simulink model "First_HIL_Scenario2"  (R2023a)
settings: Solver=ode1  StartTime=0.0  StopTime=inf  FixedStep=0.001  RelTol=1e-3
undefined symbols (not defined in the file or in its folder): ACC_X, ACC_Y, ACC_Z, Altitude, distance, GetTimeDemo, Gyro_X, Gyro_Y, Gyro_Z, Heading, Lane_Car_Distance_Left, Lane_Car_Distance_Right, Lane_Class, Lane_Coefficient_C0, Lane_Coefficient_C1, Lane_Coefficient_C2, Lane_Coefficient_C3, Lane_Curvature, Lane_Distance, Lane_ID, Latitude, Longitude, OBJ_Class, OBJ_Height, OBJ_ID, OBJ_Length, OBJ_RCS, OBJ_S_Azimuth, OBJ_S_Elevation, OBJ_S_Range, OBJ_S_Velocity, OBJ_Velocity, OBJ_Width, OBJ_X, OBJ_Y, OBJ_Z, Pitch, Roll, Subsystem, time, Timestamp, TrafficLight_Direction, TrafficLight_State, TrafficLight_Timer, Velocity, width, x, x1, x2, x3, x4, y, y1, y2, y3, y4, Yaw
(part 3 of 4)

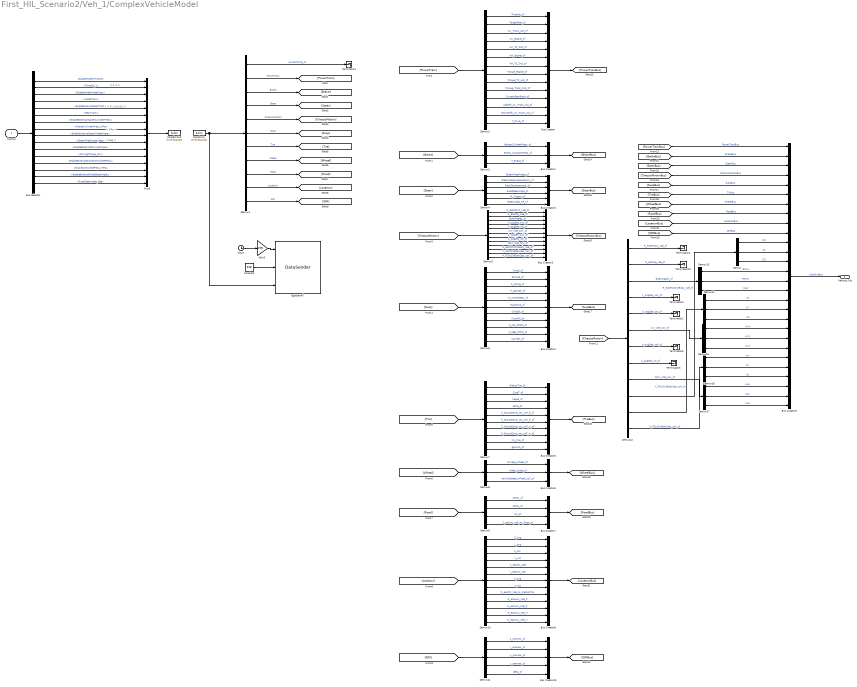
== system First_HIL_Scenario2/Veh_1/ComplexVehicleModel ==
  note: /* MPa */
  note: /* R:-1,N:0,D:1 */
  note: /* 0~1 */
  note: /* Deg */
  Control : Inport
  Bus Creator : BusCreator  Inputs=14
  Bus Creator1 : BusCreator  Inputs=3
  Bus Creator10 : BusCreator  Inputs=5
  Bus Creator2 : BusCreator  Inputs=6
  Bus Creator3 : BusCreator  Inputs=12
  Bus Creator4 : BusCreator  Inputs=11
  Bus Creator5 : BusCreator  Inputs=10
  Bus Creator6 : BusCreator  Inputs=3
  Bus Creator7 : BusCreator  Inputs=4
  Bus Creator8 : BusCreator  Inputs=13
  Bus Creator9 : BusCreator  Inputs=28
  Bus Selector : BusSelector  OutputSignals=EnableModelThrottle,Throttle_1,EnableModelModeTrans,ModeTrans,EnableExternalGearTrans,GearTrans,EnableExternalMasterCylinderPress,MasterCylinderPress_MPa,EnableExternalSteerWheelAngle,SteerWheelAngle_deg,EnableExternalDrivingTorque,DrivingTorque_Nm,EnableExternalBrakeControlledPress,BrakeControlledPress_MPa,EnableExternalRoadSteerAngle,RoadSteerAngle_deg
  Clock : Clock
  Constant : Constant  Value=228  OutDataTypeStr=int32
  Demux{,13..17} (6 alike) : Demux  Outputs=3
  Demux1 : Demux  Outputs=[1 17 9 15 36 42 36 12 16 39 5]
  Demux10 : Demux  Outputs=[1 1 4 4 4 4 1 4 4 3 3 3 3]
  Demux11 : Demux  Outputs=[1 1 1 1 1]
  Demux12 : Demux  Outputs=[3 3 3 3 3 3 3 3 3 3 3 3]
  Demux2 : Demux  Outputs=[1 1 1 1 1 1 1 1 1 1 1 1 1 4]
  Demux3 : Demux  Outputs=[1 4 4]
  Demux4 : Demux  Outputs=[1 1 1 4 4 4]
  Demux5 : Demux  Outputs=[3 3 3 3 3 3 3 3 3 3 3 3]
  Demux6 : Demux  Outputs=[4 4 4 4 2 4 4 4 4 4 4]
  Demux7 : Demux  Outputs=[4 4 4 4 3 3 3 3 4 4]
  Demux8 : Demux  Outputs=[4 4 4]
  Demux9 : Demux  Outputs=[4 4 4 4]
  EgoDataAll : S-Function  FunctionName=DataSender  Parameters='ego_all','time@i,228@[,data@d','0.01','0.0','192.168.2.101','25004'  SFunctionDeploymentMode=off  EnableBusSupport=off
  Gain3 : Gain  Gain=1000  OutDataTypeStr=Inherit: Inherit via back propagation  RndMeth=Nearest
  Mux5 : Mux  Inputs=16
  PanoSimIn : S-Function  Priority=1  FunctionName=NIVeriStandIO  Parameters=width dtype portnum stime stype btype  SFunctionDeploymentMode=off  EnableBusSupport=off  mask(NI VeriStand Inport){portnum=1, width=-1, stime=-1, dtype=auto, stype=auto, btype=1}
      mask prompts: portnum "Port number:"; width "Port dimensions (-1 for dynamically sized):"; stime "Sample time (-1 for inherited):"; dtype "Data type:"; stype "Signal type:"; btype "Block type:"
      mask help: Use this inport on any level of nested subsystems to allow NI VeriStand software to map signals to it.
      mask init:
      | NIVeriStandIO_init;
      settings: CopyFcn=NIVeriStand_MDL_functions('', 'IO_copy');  DeleteFcn=NIVeriStand_MDL_functions('', 'IO_delete');  MoveFcn=set_param(gcb, 'Mask', 'on');
      mask Callback portnum: NIVeriStand_MDL_functions('', 'IO_setportnum');
      mask TypeOptions dtype: auto | double | single | int8 | uint8 | int16 | uint16 | int32 | uint32 | boolean
      mask Callback dtype: NIVeriStand_MDL_functions('', 'IO_booleansignal');
      mask TypeOptions stype: auto | real | complex
      mask Display:
      | patch([-x x], [-y y], [.90980 .81960 .32156]);
      | plot([xrad -x x xrad], [yrad -y y yrad]);
      | fprintf('NI In%d', portnum);
  PanoSimOut : S-Function  Priority=1  FunctionName=NIVeriStandIO  Parameters=width dtype portnum stime stype btype  SFunctionDeploymentMode=off  EnableBusSupport=off  mask(NI VeriStand Outport){portnum=1, width=-1, stime=-1, dtype=auto, stype=auto, btype=0}
      mask prompts: portnum "Port number:"; width "Port dimensions (-1 for dynamically sized):"; stime "Sample time (-1 for inherited):"; dtype "Data type:"; stype "Signal type:"; btype "Block type:"
      mask help: Use this outport on any level of nested subsystems to allow NI VeriStand software to map signals to it.
      mask init:
      | NIVeriStandIO_init;
      settings: CopyFcn=NIVeriStand_MDL_functions('', 'IO_copy');  DeleteFcn=NIVeriStand_MDL_functions('', 'IO_delete');  MoveFcn=set_param(gcb, 'Mask', 'on');
      mask Callback portnum: NIVeriStand_MDL_functions('', 'IO_setportnum');
      mask TypeOptions dtype: auto | double | single | int8 | uint8 | int16 | uint16 | int32 | uint32 | boolean
      mask Callback dtype: NIVeriStand_MDL_functions('', 'IO_booleansignal');
      mask TypeOptions stype: auto | real | complex
      mask Display:
      | patch([-x x], [-y y], [.90980 .81960 .32156]);
      | plot([xrad -x x xrad], [yrad -y y yrad]);
      | fprintf('NI Out%d', portnum);
  Terminator{1..6,20} (7 alike) : Terminator
  Vehicle_Out : Outport
  wires:
  Demux12/4 -> Terminator5/1  "V_scg2eo_coV_sf"
  Demux12/7 -> Terminator6/1  "A_scg2eo_coV_sf"
  Demux12/12 -> Demux16/1  "A_FCtcCinBody2eo_coV_sf"
  Demux12/1 -> Terminator4/1  "R_eo2FCtcC_coE_sf"
  Demux12/11 -> Demux14/1  "V_FCtcCinBody2eo_coV_sf"
  Demux12/10 -> Demux/1  "R_eo2FCtcCinBody_coE_sf"
  Demux12/9 -> Demux17/1  "DAV_V2E_coV_sf"
  Demux12/8 -> Terminator3/1  "A_acg2eo_coI_sf"
  Demux12/3 -> Demux13/1  "EulerAngles_sf"
  Demux12/6 -> Demux15/1  "AV_V2E_coV_sf"
  Demux12/2 -> Terminator20/1  "R_eo2scg_coE_sf"
  Demux12/5 -> Terminator2/1  "V_acg2eo_coI_sf"
  [ChassisMotion] -> Demux12/1
  Demux5/10 -> Bus Creator3/10  "R_eo2FCtcCinBody_coE_sf"
  Demux5/6 -> Bus Creator3/6  "AV_V2E_coV_sf"
  Demux5/3 -> Bus Creator3/3  "EulerAngles_sf"
  Demux5/1 -> Bus Creator3/1  "R_eo2FCtcC_coE_sf"
  Demux5/5 -> Bus Creator3/5  "V_acg2eo_coI_sf"
  Demux5/9 -> Bus Creator3/9  "DAV_V2E_coV_sf"
  Demux5/11 -> Bus Creator3/11  "V_FCtcCinBody2eo_coV_sf"
  Demux5/7 -> Bus Creator3/7  "A_scg2eo_coV_sf"
  Demux5/8 -> Bus Creator3/8  "A_acg2eo_coI_sf"
  Demux5/4 -> Bus Creator3/4  "V_scg2eo_coV_sf"
  Demux5/2 -> Bus Creator3/2  "R_eo2scg_coE_sf"
  Demux5/12 -> Bus Creator3/12  "A_FCtcCinBody2eo_coV_sf"
  Bus Creator3/1 -> [ChassisMotionBus]
  [ChassisMotion] -> Demux5/1
  Demux17/3 -> Bus Creator9/28  "AAz"
  Demux17/2 -> Bus Creator9/27  "AAy"
  Demux17/1 -> Bus Creator9/26  "AAx"
  Demux16/3 -> Bus Creator9/25  "Az"
  Demux16/2 -> Bus Creator9/24  "Ay"
  Demux16/1 -> Bus Creator9/23  "Ax"
  Demux15/3 -> Bus Creator9/22  "AVz"
  Demux15/2 -> Bus Creator9/21  "AVy"
  Demux15/1 -> Bus Creator9/20  "AVx"
  Demux14/3 -> Bus Creator9/19  "VZ"
  Demux14/2 -> Bus Creator9/18  "VY"
  Demux14/1 -> Bus Creator9/17  "VX"
  Demux13/3 -> Bus Creator9/16  "YAW"
  Demux13/2 -> Bus Creator9/15  "PITCH"
  Demux13/1 -> Bus Creator9/14  "ROLL"
  Demux/3 -> Bus Creator9/13  "ZO"
  Demux/2 -> Bus Creator9/12  "YO"
  Demux/1 -> Bus Creator9/11  "XO"
  Demux10/10 -> Bus Creator8/10  "R_eo2uwc_coE_fl"
  Demux6/10 -> Bus Creator4/10  "F_REB_STOP_sf"
  Demux2/9 -> Bus Creator/9  "Torque_TC_out_sf"
  [TireBus] -> Bus Creator9/6  "TirBus"
  Demux4/1 -> Bus Creator2/1  "SteerWheelAngle_sf"
  Demux6/9 -> Bus Creator4/9  "F_JNC_STOP_sf"
  Demux7/6 -> Bus Creator5/6  "F_Ground2tire_ctc_coT_fr_sf"
  Demux2/2 -> Bus Creator/2  "TargetGear_sf"
  Demux9/1 -> Bus Creator7/1  "DZDX_sf"
  [WheelBus] -> Bus Creator9/7  "WheelBus"
  Bus Creator5/1 -> [TireBus]
  Demux7/3 -> Bus Creator5/3  "kappa_sf"
  Demux6/2 -> Bus Creator4/2  "DCmpS_sf"
  Demux7/10 -> Bus Creator5/10  "gamma_sf"
  Bus Creator1/1 -> [BrakeBus]
  Demux4/4 -> Bus Creator2/4  "RoadSteerAngle_sf"
  Demux7/1 -> Bus Creator5/1  "RadiusTire_sf"
  Demux6/11 -> Bus Creator4/11  "Camber_sf"
  Demux4/6 -> Bus Creator2/6  "SteerAngle_KP_sf"
  [Steer] -> Demux4/1
  [BrakeBus] -> Bus Creator9/2  "BrakeBus"
  Demux10/5 -> Bus Creator8/5  "X_eo2ctc_coE"
  Demux6/8 -> Bus Creator4/8  "CmpRSt_sf"
  Demux8/2 -> Bus Creator6/2  "wheel_state_sf"
  Bus Creator7/1 -> [RoadBus]
  Demux2/6 -> Bus Creator/6  "AA_Engine_sf"
  Bus Creator9/1 -> Vehicle_Out/1  "xCarOutBus"
  Demux6/6 -> Bus Creator4/6  "SuspCmp_sf"
  Demux7/7 -> Bus Creator5/7  "F_Ground2tire_ctc_coT_rl_sf"
  Demux2/1 -> Bus Creator/1  "Throttle_sf"
  Demux6/3 -> Bus Creator4/3  "F_spring_sf"
  Demux10/12 -> Bus Creator8/12  "R_eo2uwc_coE_rl"
  Demux4/5 -> Bus Creator2/5  "M_Kingpin_sf"
  Bus Creator10/1 -> [IDMBus]
  Demux2/13 -> Bus Creator/13  "DownShift_AV_Trans_out_sf"
  [Tire] -> Demux7/1
  [PowerTrainBus] -> Bus Creator9/1  "PowerTrainBus"
  Demux3/2 -> Bus Creator1/2  "Brake_ActuatorPress_sf"
  Demux9/2 -> Bus Creator7/2  "DZDY_sf"
  Bus Creator4/1 -> [SuspBus]
  Demux7/9 -> Bus Creator5/9  "My_tire_sf"
  Demux6/5 -> Bus Creator4/5  "M_AntiRollBar_sf"
  Bus Creator/1 -> [PowerTrainBus]
  Demux3/3 -> Bus Creator1/3  "T_Brake_sf"
  Demux2/7 -> Bus Creator/7  "AA_TC_Out_sf"
  Demux2/10 -> Bus Creator/10  "Torque_Trans_Out_sf"
  [PowerTrain] -> Demux2/1
  Demux2/12 -> Bus Creator/12  "UpShift_AV_Trans_out_sf"
  [LocationBus] -> Bus Creator9/9  "LocationBus"
  Demux2/14 -> Bus Creator/14  "T_Drive_sf"
  Demux4/3 -> Bus Creator2/3  "RackDisplacement_sf"
  Demux2/8 -> Bus Creator/8  "Torque_Engine_sf"
  Demux3/1 -> Bus Creator1/1  "MasterCylinderPress_sf"
  [Brake] -> Demux3/1
  Demux10/13 -> Bus Creator8/13  "R_eo2uwc_coE_rr"
  Demux6/4 -> Bus Creator4/4  "F_damper_sf"
  Demux7/2 -> Bus Creator5/2  "CmpT_sf"
  Demux8/3 -> Bus Creator6/3  "VerticalSpeed_Wheel_coV_sf"
  Demux7/5 -> Bus Creator5/5  "F_Ground2tire_ctc_coT_fl_sf"
  Demux9/3 -> Bus Creator7/3  "mu_sf"
  [Road] -> Demux9/1
  Demux7/8 -> Bus Creator5/8  "F_Ground2tire_ctc_coT_rr_sf"
  [Wheel] -> Demux8/1
  Demux8/1 -> Bus Creator6/1  "Omega_Wheel_sf"
  Demux10/2 -> Bus Creator8/2  "L_scg"
  Demux4/2 -> Bus Creator2/2  "SteerWheelAngleVelocity_sf"
  Demux2/11 -> Bus Creator/11  "CurrentGearRatio_sf"
  Bus Creator8/1 -> [LocationBus]
  Demux10/1 -> Bus Creator8/1  "S_scg"
  [Location] -> Demux10/1
  Demux7/4 -> Bus Creator5/4  "alpha_sf"
  Bus Creator2/1 -> [SteerBus]
  Demux2/4 -> Bus Creator/4  "AV_Engine_sf"
  Demux10/3 -> Bus Creator8/3  "S_ctc"
  Demux10/4 -> Bus Creator8/4  "L_ctc"
  Demux2/3 -> Bus Creator/3  "AV_Trans_out_sf"
  Bus Creator6/1 -> [WheelBus]
  Demux11/1 -> Bus Creator10/1  "s_preview_sf"
  Demux10/7 -> Bus Creator8/7  "k_scg"
  [ChassisMotionBus] -> Bus Creator9/4  "ChassisMotionBus"
  Demux2/5 -> Bus Creator/5  "AV_TC_Out_sf"
  [SuspBus] -> Bus Creator9/5  "SuspBus"
  Demux10/8 -> Bus Creator8/8  "k_ctc"
  [IDM] -> Demux11/1
  [SteerBus] -> Bus Creator9/3  "SteerBus"
  Demux11/2 -> Bus Creator10/2  "l_preview_sf"
  Demux9/4 -> Bus Creator7/4  "Z_eo2ctc_coE_by_Road_sf"
  Demux11/3 -> Bus Creator10/3  "x_preview_sf"
  Demux6/1 -> Bus Creator4/1  "CmpS_sf"
  Demux6/7 -> Bus Creator4/7  "CmpJSt_sf"
  [IDMBus] -> Bus Creator9/10  "IDMBus"
  Demux11/5 -> Bus Creator10/5  "delta_sf"
  [RoadBus] -> Bus Creator9/8  "RoadBus"
  [Susp] -> Demux6/1
  Demux10/6 -> Bus Creator8/6  "Y_eo2ctc_coE"
  Demux10/9 -> Bus Creator8/9  "Z_eo2ctc_coE_by_RadiusTire"
  Demux11/4 -> Bus Creator10/4  "y_preview_sf"
  Demux10/11 -> Bus Creator8/11  "R_eo2uwc_coE_fr"
  Demux1/10 -> [Location]  "Location"
  Demux1/2 -> [PowerTrain]  "PowerTrain"
  Demux1/11 -> [IDM]  "IDM"
  Demux1/3 -> [Brake]  "Brake"
  PanoSimIn/1 -> EgoDataAll/3, Demux1/1
  Demux1/6 -> [Susp]  "Susp"
  Demux1/1 -> Terminator1/1  "currentTime_sf"
  Demux1/9 -> [Road]  "Road"
  Demux1/5 -> [ChassisMotion]  "ChassisMotion"
  Demux1/7 -> [Tire]  "Tire"
  Demux1/8 -> [Wheel]  "Wheel"
  Demux1/4 -> [Steer]  "Steer"
  Bus Selector/16 -> Mux5/16  "<RoadSteerAngle_deg>"
  Bus Selector/15 -> Mux5/15  "<EnableExternalRoadSteerAngle>"
  Bus Selector/9 -> Mux5/9  "<EnableExternalSteerWheelAngle>"
  Bus Selector/7 -> Mux5/7  "<EnableExternalMasterCylinderPress>"
  Control/1 -> Bus Selector/1
  Bus Selector/14 -> Mux5/14  "<BrakeControlledPress_MPa>"
  Bus Selector/3 -> Mux5/3  "<EnableModelModeTrans>"
  Bus Selector/8 -> Mux5/8  "<MasterCylinderPress_MPa>"
  Bus Selector/11 -> Mux5/11  "<EnableExternalDrivingTorque>"
  Bus Selector/2 -> Mux5/2  "<Throttle_1>"
  Bus Selector/1 -> Mux5/1  "<EnableModelThrottle>"
  Bus Selector/5 -> Mux5/5  "<EnableExternalGearTrans>"
  Bus Selector/6 -> Mux5/6  "<GearTrans>"
  Bus Selector/4 -> Mux5/4  "<ModeTrans>"
  Bus Selector/12 -> Mux5/12  "<DrivingTorque_Nm>"
  Bus Selector/13 -> Mux5/13  "<EnableExternalBrakeControlledPress>"
  Bus Selector/10 -> Mux5/10  "<SteerWheelAngle_deg>"
  Mux5/1 -> PanoSimOut/1
  Constant/1 -> EgoDataAll/2
  Gain3/1 -> EgoDataAll/1
  Clock/1 -> Gain3/1

== system First_HIL_Scenario2/Veh_1/DriverModel ==
  In1 : Inport
  DriverFilter : Subsystem
  DriverOut : Outport
  wires:
  DriverFilter/1(DriverOut) -> DriverOut/1

== system First_HIL_Scenario2/Veh_1/GlobalVariable ==
  Bus Creator : BusCreator  Inputs=2
  variable : Subsystem
  Value : Outport
  Original : Outport  Port=2
  wires:
  Bus Creator/1 -> Original/1
  variable/2(Out2) -> Bus Creator/2  "Time"
  variable/1(Out1) -> Value/1, Bus Creator/1  "Value"

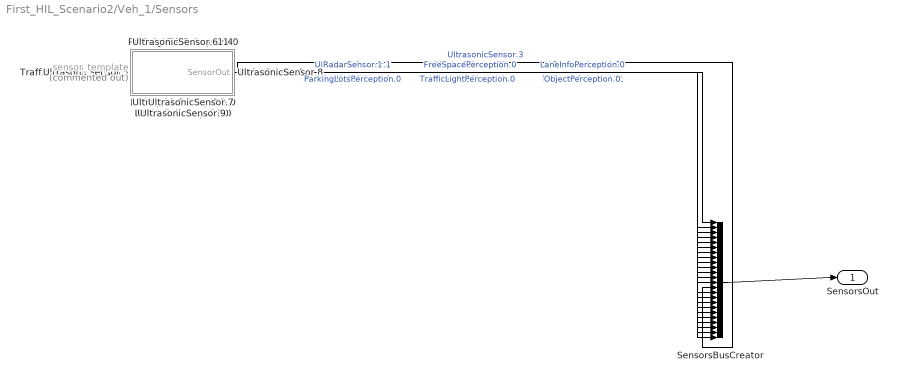
== system First_HIL_Scenario2/Veh_1/Sensors ==
  FreeSpacePerception.0 : Subsystem
  GNSS.0 : Subsystem
  IMU.0 : Subsystem
  LaneInfoPerception.0 : Subsystem
  ObjectPerception.0 : Subsystem
  ParkingLotsPerception.0 : Subsystem
  RadarSensor.0 : Subsystem
  RadarSensor.1 : Subsystem
  RadarSensor.2 : Subsystem
  RadarSensor.3 : Subsystem
  RadarSensor.4 : Subsystem
  SensorsBusCreator : BusCreator  Inputs=FreeSpacePerception.0,LaneInfoPerception.0,ObjectPerception.0,ParkingLotsPerception.0,TrafficLightPerception.0,RadarSensor.0,RadarSensor.1,RadarSensor.2,RadarSensor.3,RadarSensor.4,UltrasonicSensor.0,UltrasonicSensor.1,UltrasonicSensor.2,UltrasonicSensor.3,UltrasonicSensor.4,UltrasonicSensor.5,UltrasonicSensor.6,UltrasonicSensor.7,UltrasonicSensor.8,UltrasonicSensor.9,UltrasonicSensor.10,UltrasonicSensor.11,GNSS.0,IMU.0
  TrafficLightPerception.0 : Subsystem
  UltrasonicSensor.0 : Subsystem
  UltrasonicSensor.1 : Subsystem
  UltrasonicSensor.10 : Subsystem
  UltrasonicSensor.11 : Subsystem
  UltrasonicSensor.2 : Subsystem
  UltrasonicSensor.3 : Subsystem
  UltrasonicSensor.4 : Subsystem
  UltrasonicSensor.5 : Subsystem
  UltrasonicSensor.6 : Subsystem
  UltrasonicSensor.7 : Subsystem
  UltrasonicSensor.8 : Subsystem
  UltrasonicSensor.9 : Subsystem
  sensor_template : Subsystem  Commented=on
  SensorsOut : Outport
  wires:
  SensorsBusCreator/1 -> SensorsOut/1
  IMU.0/1(SensorOut) -> SensorsBusCreator/24  "IMU.0"
  GNSS.0/1(SensorOut) -> SensorsBusCreator/23  "GNSS.0"
  UltrasonicSensor.11/1(SensorOut) -> SensorsBusCreator/22  "UltrasonicSensor.11"
  UltrasonicSensor.10/1(SensorOut) -> SensorsBusCreator/21  "UltrasonicSensor.10"
  UltrasonicSensor.9/1(SensorOut) -> SensorsBusCreator/20  "UltrasonicSensor.9"
  UltrasonicSensor.8/1(SensorOut) -> SensorsBusCreator/19  "UltrasonicSensor.8"
  UltrasonicSensor.7/1(SensorOut) -> SensorsBusCreator/18  "UltrasonicSensor.7"
  UltrasonicSensor.6/1(SensorOut) -> SensorsBusCreator/17  "UltrasonicSensor.6"
  UltrasonicSensor.5/1(SensorOut) -> SensorsBusCreator/16  "UltrasonicSensor.5"
  UltrasonicSensor.4/1(SensorOut) -> SensorsBusCreator/15  "UltrasonicSensor.4"
  UltrasonicSensor.3/1(SensorOut) -> SensorsBusCreator/14  "UltrasonicSensor.3"
  UltrasonicSensor.2/1(SensorOut) -> SensorsBusCreator/13  "UltrasonicSensor.2"
  UltrasonicSensor.1/1(SensorOut) -> SensorsBusCreator/12  "UltrasonicSensor.1"
  UltrasonicSensor.0/1(SensorOut) -> SensorsBusCreator/11  "UltrasonicSensor.0"
  RadarSensor.4/1(SensorOut) -> SensorsBusCreator/10  "RadarSensor.4"
  RadarSensor.3/1(SensorOut) -> SensorsBusCreator/9  "RadarSensor.3"
  RadarSensor.2/1(SensorOut) -> SensorsBusCreator/8  "RadarSensor.2"
  RadarSensor.1/1(SensorOut) -> SensorsBusCreator/7  "RadarSensor.1"
  RadarSensor.0/1(SensorOut) -> SensorsBusCreator/6  "RadarSensor.0"
  TrafficLightPerception.0/1(SensorOut) -> SensorsBusCreator/5  "TrafficLightPerception.0"
  ParkingLotsPerception.0/1(SensorOut) -> SensorsBusCreator/4  "ParkingLotsPerception.0"
  ObjectPerception.0/1(SensorOut) -> SensorsBusCreator/3  "ObjectPerception.0"
  LaneInfoPerception.0/1(SensorOut) -> SensorsBusCreator/2  "LaneInfoPerception.0"
  FreeSpacePerception.0/1(SensorOut) -> SensorsBusCreator/1  "FreeSpacePerception.0"

== system First_HIL_Scenario2/Veh_1/VehicleDataBus ==
  VehicleDynOut : Inport
  GlobalVariable : Inport  Port=2
  GlobalVariableOriginal : Inport  Port=3
  Clock : Clock
  EgoBus : Subsystem
  EgoExtraBus : Subsystem
  Gain3 : Gain  Gain=1000  OutDataTypeStr=Inherit: Inherit via back propagation  RndMeth=Nearest
  GlobalVariableWrite : Subsystem
  wires:
  GlobalVariableWrite/1(Out1) -> EgoBus/3(VehiclleDyn1)
  EgoExtraBus/1(Out1) -> EgoBus/4(VehiclleDyn2)
  Gain3/1 -> EgoExtraBus/1(clock), EgoBus/1(clock), GlobalVariableWrite/3(In3)
  GlobalVariableOriginal/1 -> GlobalVariableWrite/2(In2)
  GlobalVariable/1 -> GlobalVariableWrite/1(In1)
  Clock/1 -> Gain3/1
  VehicleDynOut/1 -> EgoExtraBus/2(VehiclleDyn), EgoBus/2(VehiclleDyn)

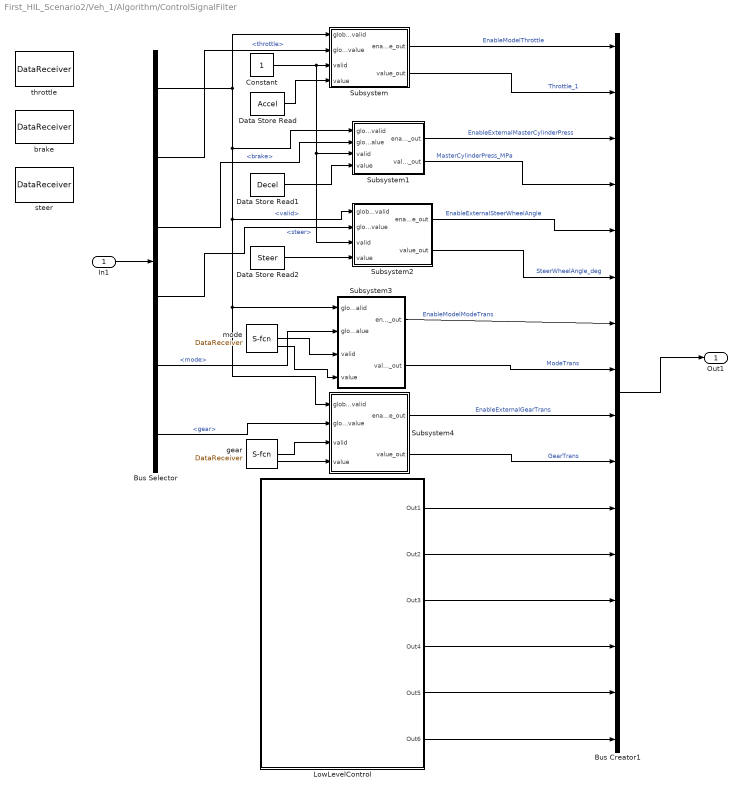
== system First_HIL_Scenario2/Veh_1/Algorithm/ControlSignalFilter ==
  In1 : Inport
  Bus Creator1 : BusCreator  Inputs=16
  Bus Selector : BusSelector  OutputSignals=valid,throttle,brake,steer,mode,gear
  Constant : Constant
  Data Store Read : DataStoreRead  DataStoreName=Accel  IndexOptions=Index vector (dialog)  Indices=1  OutputSizes=1
  Data Store Read1 : DataStoreRead  DataStoreName=Decel  IndexOptions=Index vector (dialog)  Indices=1  OutputSizes=1
  Data Store Read2 : DataStoreRead  DataStoreName=Steer  IndexOptions=Index vector (dialog)  Indices=1  OutputSizes=1
  LowLevelControl : Subsystem  AncestorBlock=GetTimeDemo/Subsystem
  Subsystem : Subsystem
  Subsystem1 : Subsystem
  Subsystem2 : Subsystem
  Subsystem3 : Subsystem
  Subsystem4 : Subsystem
  brake : S-Function  FunctionName=DataReceiver  Parameters='ego_control.brake','time@i,valid@b,brake@d','0.001','0.0','192.168.2.195','25003'  SFunctionDeploymentMode=off  EnableBusSupport=off
  gear : S-Function  FunctionName=DataReceiver  Parameters='ego_control.gear','time@i,valid@b,gear@i','0.001','0.0','192.168.2.195','25006'  SFunctionDeploymentMode=off  EnableBusSupport=off
  mode : S-Function  FunctionName=DataReceiver  Parameters='ego_control.mode','time@i,valid@b,mode@i','0.001','0.0','192.168.2.195','25005'  SFunctionDeploymentMode=off  EnableBusSupport=off
  steer : S-Function  FunctionName=DataReceiver  Parameters='ego_control.steer','time@i,valid@b,steer@d','0.001','0.0','192.168.2.195','25004'  SFunctionDeploymentMode=off  EnableBusSupport=off
  throttle : S-Function  FunctionName=DataReceiver  Parameters='ego_control.throttle','time@i,valid@b,throttle@d','0.001','0.0','192.168.2.195','25002'  SFunctionDeploymentMode=off  EnableBusSupport=off
  Out1 : Outport
  wires:
  In1/1 -> Bus Selector/1
  Bus Selector/2 -> Subsystem/2(global_value)  "<throttle>"
  Bus Creator1/1 -> Out1/1
  Subsystem1/2(value_out) -> Bus Creator1/4  "MasterCylinderPress_MPa"
  Bus Selector/3 -> Subsystem1/2(global_value)  "<brake>"
  Subsystem2/2(value_out) -> Bus Creator1/6  "SteerWheelAngle_deg"
  Bus Selector/4 -> Subsystem2/2(global_value)  "<steer>"
  Bus Selector/1 -> Subsystem/1(global_valid), Subsystem4/1(global_valid), Subsystem3/1(global_valid), Subsystem2/1(global_valid), Subsystem1/1(global_valid)  "<valid>"
  Subsystem/1(enable_out) -> Bus Creator1/1  "EnableModelThrottle"
  Subsystem/2(value_out) -> Bus Creator1/2  "Throttle_1"
  Subsystem1/1(enable_out) -> Bus Creator1/3  "EnableExternalMasterCylinderPress"
  Subsystem2/1(enable_out) -> Bus Creator1/5  "EnableExternalSteerWheelAngle"
  Bus Selector/5 -> Subsystem3/2(global_value)  "<mode>"
  Bus Selector/6 -> Subsystem4/2(global_value)  "<gear>"
  Subsystem3/1(enable_out) -> Bus Creator1/7  "EnableModelModeTrans"
  Subsystem3/2(value_out) -> Bus Creator1/8  "ModeTrans"
  Subsystem4/1(enable_out) -> Bus Creator1/9  "EnableExternalGearTrans"
  Subsystem4/2(value_out) -> Bus Creator1/10  "GearTrans"
  mode/2 -> Subsystem3/3(valid)
  mode/3 -> Subsystem3/4(value)
  gear/2 -> Subsystem4/3(valid)
  gear/3 -> Subsystem4/4(value)
  LowLevelControl/1(Out1) -> Bus Creator1/11
  LowLevelControl/2(Out2) -> Bus Creator1/12
  LowLevelControl/3(Out3) -> Bus Creator1/13
  LowLevelControl/4(Out4) -> Bus Creator1/14
  LowLevelControl/5(Out5) -> Bus Creator1/15
  LowLevelControl/6(Out6) -> Bus Creator1/16
  Constant/1 -> Subsystem1/3(valid), Subsystem2/3(valid), Subsystem/3(valid)
  Data Store Read/1 -> Subsystem/4(value)
  Data Store Read1/1 -> Subsystem1/4(value)
  Data Store Read2/1 -> Subsystem2/4(value)

== system First_HIL_Scenario2/Veh_1/DriverModel/DriverFilter ==
  note: DriverBusCreator
  Bus Creator2 : BusCreator  Inputs=6
  EgoControlBus : S-Function  FunctionName=DataReceiver  Parameters='ego_control','time@i,valid@b,throttle@d,brake@d,steer@d,mode@i,gear@i','0.001','0.0','192.168.2.195','25001'  SFunctionDeploymentMode=off  EnableBusSupport=off
  DriverOut : Outport
  wires:
  EgoControlBus/7 -> Bus Creator2/6  "gear"
  EgoControlBus/6 -> Bus Creator2/5  "mode"
  EgoControlBus/2 -> Bus Creator2/1  "valid"
  EgoControlBus/3 -> Bus Creator2/2  "throttle"
  EgoControlBus/5 -> Bus Creator2/4  "steer"
  EgoControlBus/4 -> Bus Creator2/3  "brake"
  Bus Creator2/1 -> DriverOut/1

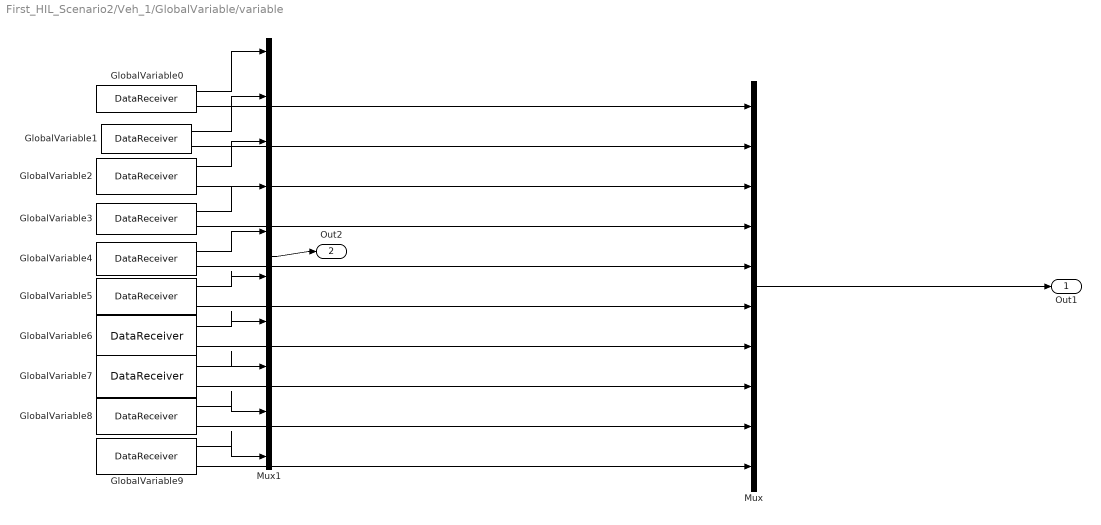
== system First_HIL_Scenario2/Veh_1/GlobalVariable/variable ==
  GlobalVariable0 : S-Function  FunctionName=DataReceiver  Parameters='global.0','time@i,variable@d','0.01','0.0','192.168.2.195','25010'  SFunctionDeploymentMode=off  EnableBusSupport=off
  GlobalVariable1 : S-Function  FunctionName=DataReceiver  Parameters='global.1','time@i,variable@d','0.01','0.0','192.168.2.195','25011'  SFunctionDeploymentMode=off  EnableBusSupport=off
  GlobalVariable2 : S-Function  FunctionName=DataReceiver  Parameters='global.2','time@i,variable@d','0.01','0.0','192.168.2.195','25012'  SFunctionDeploymentMode=off  EnableBusSupport=off
  GlobalVariable3 : S-Function  FunctionName=DataReceiver  Parameters='global.3','time@i,variable@d','0.01','0.0','192.168.2.195','25013'  SFunctionDeploymentMode=off  EnableBusSupport=off
  GlobalVariable4 : S-Function  FunctionName=DataReceiver  Parameters='global.4','time@i,variable@d','0.01','0.0','192.168.2.195','25014'  SFunctionDeploymentMode=off  EnableBusSupport=off
  GlobalVariable5 : S-Function  FunctionName=DataReceiver  Parameters='global.5','time@i,variable@d','0.01','0.0','192.168.2.195','25015'  SFunctionDeploymentMode=off  EnableBusSupport=off
  GlobalVariable6 : S-Function  FunctionName=DataReceiver  Parameters='global.6','time@i,variable@d','0.01','0.0','192.168.2.195','25016'  SFunctionDeploymentMode=off  EnableBusSupport=off
  GlobalVariable7 : S-Function  FunctionName=DataReceiver  Parameters='global.7','time@i,variable@d','0.01','0.0','192.168.2.195','25017'  SFunctionDeploymentMode=off  EnableBusSupport=off
  GlobalVariable8 : S-Function  FunctionName=DataReceiver  Parameters='global.8','time@i,variable@d','0.01','0.0','192.168.2.195','25018'  SFunctionDeploymentMode=off  EnableBusSupport=off
  GlobalVariable9 : S-Function  FunctionName=DataReceiver  Parameters='global.9','time@i,variable@d','0.01','0.0','192.168.2.195','25019'  SFunctionDeploymentMode=off  EnableBusSupport=off
  Mux : Mux  Inputs=10
  Mux1 : Mux  Inputs=10
  Out1 : Outport
  Out2 : Outport  Port=2
  wires:
  GlobalVariable2/1 -> Mux1/3
  GlobalVariable8/1 -> Mux1/9
  GlobalVariable9/1 -> Mux1/10
  GlobalVariable7/1 -> Mux1/8
  GlobalVariable6/1 -> Mux1/7
  GlobalVariable5/1 -> Mux1/6
  GlobalVariable4/1 -> Mux1/5
  GlobalVariable3/1 -> Mux1/4
  GlobalVariable0/1 -> Mux1/1
  GlobalVariable1/1 -> Mux1/2
  GlobalVariable9/2 -> Mux/10
  GlobalVariable8/2 -> Mux/9
  GlobalVariable7/2 -> Mux/8
  GlobalVariable6/2 -> Mux/7
  GlobalVariable5/2 -> Mux/6
  GlobalVariable4/2 -> Mux/5
  GlobalVariable3/2 -> Mux/4
  GlobalVariable2/2 -> Mux/3
  GlobalVariable1/2 -> Mux/2
  GlobalVariable0/2 -> Mux/1
  Mux1/1 -> Out2/1
  Mux/1 -> Out1/1

== system First_HIL_Scenario2/Veh_1/Sensors/FreeSpacePerception.0 ==
  BusCreator : BusCreator  Inputs=time,width,x,y
  SensorBus : S-Function  FunctionName=DataReceiver  Parameters='FreeSpacePerception.0','time@i,36000@[,x@d,y@d','0.01','0.0','192.168.2.195','25100'  SFunctionDeploymentMode=off  EnableBusSupport=off
  SensorOut : Outport
  wires:
  SensorBus/4 -> BusCreator/4  "y"
  SensorBus/3 -> BusCreator/3  "x"
  SensorBus/2 -> BusCreator/2  "width"
  SensorBus/1 -> BusCreator/1  "time"
  BusCreator/1 -> SensorOut/1

== system First_HIL_Scenario2/Veh_1/Sensors/GNSS.0 ==
  BusCreator : BusCreator  Inputs=Timestamp,Longitude,Latitude,Altitude,Heading,Velocity
  SensorBus : S-Function  FunctionName=DataReceiver  Parameters='GNSS.0','Timestamp@i,Longitude@d,Latitude@d,Altitude@d,Heading@d,Velocity@d','0.01','0.0','192.168.2.195','25127'  SFunctionDeploymentMode=off  EnableBusSupport=off
  SensorOut : Outport
  wires:
  SensorBus/6 -> BusCreator/6  "Velocity"
  SensorBus/5 -> BusCreator/5  "Heading"
  SensorBus/4 -> BusCreator/4  "Altitude"
  SensorBus/3 -> BusCreator/3  "Latitude"
  SensorBus/2 -> BusCreator/2  "Longitude"
  SensorBus/1 -> BusCreator/1  "Timestamp"
  BusCreator/1 -> SensorOut/1

== system First_HIL_Scenario2/Veh_1/Sensors/IMU.0 ==
  BusCreator : BusCreator  Inputs=Timestamp,ACC_X,ACC_Y,ACC_Z,Gyro_X,Gyro_Y,Gyro_Z,Yaw,Pitch,Roll
  SensorBus : S-Function  FunctionName=DataReceiver  Parameters='IMU.0','Timestamp@i,ACC_X@d,ACC_Y@d,ACC_Z@d,Gyro_X@d,Gyro_Y@d,Gyro_Z@d,Yaw@d,Pitch@d,Roll@d','0.01','0.0','192.168.2.195','25128'  SFunctionDeploymentMode=off  EnableBusSupport=off
  SensorOut : Outport
  wires:
  SensorBus/10 -> BusCreator/10  "Roll"
  SensorBus/9 -> BusCreator/9  "Pitch"
  SensorBus/8 -> BusCreator/8  "Yaw"
  SensorBus/7 -> BusCreator/7  "Gyro_Z"
  SensorBus/6 -> BusCreator/6  "Gyro_Y"
  SensorBus/5 -> BusCreator/5  "Gyro_X"
  SensorBus/4 -> BusCreator/4  "ACC_Z"
  SensorBus/3 -> BusCreator/3  "ACC_Y"
  SensorBus/2 -> BusCreator/2  "ACC_X"
  SensorBus/1 -> BusCreator/1  "Timestamp"
  BusCreator/1 -> SensorOut/1

== system First_HIL_Scenario2/Veh_1/Sensors/LaneInfoPerception.0 ==
  BusCreator : BusCreator  Inputs=Timestamp,width,Lane_ID,Lane_Distance,Lane_Car_Distance_Left,Lane_Car_Distance_Right,Lane_Curvature,Lane_Coefficient_C0,Lane_Coefficient_C1,Lane_Coefficient_C2,Lane_Coefficient_C3,Lane_Class
  SensorBus : S-Function  FunctionName=DataReceiver  Parameters='LaneInfoPerception.0','Timestamp@i,4@[,Lane_ID@i,Lane_Distance@d,Lane_Car_Distance_Left@d,Lane_Car_Distance_Right@d,Lane_Curvature@d,Lane_Coefficient_C0@d,Lane_Coefficient_C1@d,Lane_Coefficient_C2@d,Lane_Coefficient_C3@d,Lane_Class@b','0.01','0.0','192.168.2.195','25101'  SFunctionDeploymentMode=off  EnableBusSupport=off
  SensorOut : Outport
  wires:
  SensorBus/12 -> BusCreator/12  "Lane_Class"
  SensorBus/11 -> BusCreator/11  "Lane_Coefficient_C3"
  SensorBus/10 -> BusCreator/10  "Lane_Coefficient_C2"
  SensorBus/9 -> BusCreator/9  "Lane_Coefficient_C1"
  SensorBus/8 -> BusCreator/8  "Lane_Coefficient_C0"
  SensorBus/7 -> BusCreator/7  "Lane_Curvature"
  SensorBus/6 -> BusCreator/6  "Lane_Car_Distance_Right"
  SensorBus/5 -> BusCreator/5  "Lane_Car_Distance_Left"
  SensorBus/4 -> BusCreator/4  "Lane_Distance"
  SensorBus/3 -> BusCreator/3  "Lane_ID"
  SensorBus/2 -> BusCreator/2  "width"
  SensorBus/1 -> BusCreator/1  "Timestamp"
  BusCreator/1 -> SensorOut/1

== system First_HIL_Scenario2/Veh_1/Sensors/ObjectPerception.0 ==
  BusCreator : BusCreator  Inputs=Timestamp,width,OBJ_ID,OBJ_Class,OBJ_X,OBJ_Y,OBJ_Z,OBJ_Velocity,OBJ_Length,OBJ_Width,OBJ_Height
  SensorBus : S-Function  FunctionName=DataReceiver  Parameters='ObjectPerception.0','Timestamp@i,64@[,OBJ_ID@i,OBJ_Class@b,OBJ_X@d,OBJ_Y@d,OBJ_Z@d,OBJ_Velocity@d,OBJ_Length@d,OBJ_Width@d,OBJ_Height@d','0.01','0.0','192.168.2.195','25102'  SFunctionDeploymentMode=off  EnableBusSupport=off
  SensorOut : Outport
  wires:
  SensorBus/11 -> BusCreator/11  "OBJ_Height"
  SensorBus/10 -> BusCreator/10  "OBJ_Width"
  SensorBus/9 -> BusCreator/9  "OBJ_Length"
  SensorBus/8 -> BusCreator/8  "OBJ_Velocity"
  SensorBus/7 -> BusCreator/7  "OBJ_Z"
  SensorBus/6 -> BusCreator/6  "OBJ_Y"
  SensorBus/5 -> BusCreator/5  "OBJ_X"
  SensorBus/4 -> BusCreator/4  "OBJ_Class"
  SensorBus/3 -> BusCreator/3  "OBJ_ID"
  SensorBus/2 -> BusCreator/2  "width"
  SensorBus/1 -> BusCreator/1  "Timestamp"
  BusCreator/1 -> SensorOut/1

== system First_HIL_Scenario2/Veh_1/Sensors/ParkingLotsPerception.0 ==
  BusCreator : BusCreator  Inputs=time,width,x1,y1,x2,y2,x3,y3,x4,y4
  SensorBus : S-Function  FunctionName=DataReceiver  Parameters='ParkingLotsPerception.0','time@i,64@[,x1@d,y1@d,x2@d,y2@d,x3@d,y3@d,x4@d,y4@d','0.01','0.0','192.168.2.195','25103'  SFunctionDeploymentMode=off  EnableBusSupport=off
  SensorOut : Outport
  wires:
  SensorBus/10 -> BusCreator/10  "y4"
  SensorBus/9 -> BusCreator/9  "x4"
  SensorBus/8 -> BusCreator/8  "y3"
  SensorBus/7 -> BusCreator/7  "x3"
  SensorBus/6 -> BusCreator/6  "y2"
  SensorBus/5 -> BusCreator/5  "x2"
  SensorBus/4 -> BusCreator/4  "y1"
  SensorBus/3 -> BusCreator/3  "x1"
  SensorBus/2 -> BusCreator/2  "width"
  SensorBus/1 -> BusCreator/1  "time"
  BusCreator/1 -> SensorOut/1

== system First_HIL_Scenario2/Veh_1/Sensors/RadarSensor.0 ==
  BusCreator : BusCreator  Inputs=time,width,OBJ_ID,OBJ_Class,OBJ_S_Azimuth,OBJ_S_Elevation,OBJ_S_Velocity,OBJ_S_Range,OBJ_RCS
  SensorBus : S-Function  FunctionName=DataReceiver  Parameters='RadarSensor.0','time@i,64@[,OBJ_ID@i,OBJ_Class@i,OBJ_S_Azimuth@d,OBJ_S_Elevation@d,OBJ_S_Velocity@d,OBJ_S_Range@d,OBJ_RCS@d','0.01','0.0','192.168.2.195','25106'  SFunctionDeploymentMode=off  EnableBusSupport=off
  SensorOut : Outport
  wires:
  SensorBus/9 -> BusCreator/9  "OBJ_RCS"
  SensorBus/8 -> BusCreator/8  "OBJ_S_Range"
  SensorBus/7 -> BusCreator/7  "OBJ_S_Velocity"
  SensorBus/6 -> BusCreator/6  "OBJ_S_Elevation"
  SensorBus/5 -> BusCreator/5  "OBJ_S_Azimuth"
  SensorBus/4 -> BusCreator/4  "OBJ_Class"
  SensorBus/3 -> BusCreator/3  "OBJ_ID"
  SensorBus/2 -> BusCreator/2  "width"
  SensorBus/1 -> BusCreator/1  "time"
  BusCreator/1 -> SensorOut/1

== system First_HIL_Scenario2/Veh_1/Sensors/RadarSensor.1 ==
  BusCreator : BusCreator  Inputs=time,width,OBJ_ID,OBJ_Class,OBJ_S_Azimuth,OBJ_S_Elevation,OBJ_S_Velocity,OBJ_S_Range,OBJ_RCS
  SensorBus : S-Function  FunctionName=DataReceiver  Parameters='RadarSensor.1','time@i,64@[,OBJ_ID@i,OBJ_Class@i,OBJ_S_Azimuth@d,OBJ_S_Elevation@d,OBJ_S_Velocity@d,OBJ_S_Range@d,OBJ_RCS@d','0.01','0.0','192.168.2.195','25107'  SFunctionDeploymentMode=off  EnableBusSupport=off
  SensorOut : Outport
  wires:
  SensorBus/9 -> BusCreator/9  "OBJ_RCS"
  SensorBus/8 -> BusCreator/8  "OBJ_S_Range"
  SensorBus/7 -> BusCreator/7  "OBJ_S_Velocity"
  SensorBus/6 -> BusCreator/6  "OBJ_S_Elevation"
  SensorBus/5 -> BusCreator/5  "OBJ_S_Azimuth"
  SensorBus/4 -> BusCreator/4  "OBJ_Class"
  SensorBus/3 -> BusCreator/3  "OBJ_ID"
  SensorBus/2 -> BusCreator/2  "width"
  SensorBus/1 -> BusCreator/1  "time"
  BusCreator/1 -> SensorOut/1

== system First_HIL_Scenario2/Veh_1/Sensors/RadarSensor.2 ==
  BusCreator : BusCreator  Inputs=time,width,OBJ_ID,OBJ_Class,OBJ_S_Azimuth,OBJ_S_Elevation,OBJ_S_Velocity,OBJ_S_Range,OBJ_RCS
  SensorBus : S-Function  FunctionName=DataReceiver  Parameters='RadarSensor.2','time@i,64@[,OBJ_ID@i,OBJ_Class@i,OBJ_S_Azimuth@d,OBJ_S_Elevation@d,OBJ_S_Velocity@d,OBJ_S_Range@d,OBJ_RCS@d','0.01','0.0','192.168.2.195','25108'  SFunctionDeploymentMode=off  EnableBusSupport=off
  SensorOut : Outport
  wires:
  SensorBus/9 -> BusCreator/9  "OBJ_RCS"
  SensorBus/8 -> BusCreator/8  "OBJ_S_Range"
  SensorBus/7 -> BusCreator/7  "OBJ_S_Velocity"
  SensorBus/6 -> BusCreator/6  "OBJ_S_Elevation"
  SensorBus/5 -> BusCreator/5  "OBJ_S_Azimuth"
  SensorBus/4 -> BusCreator/4  "OBJ_Class"
  SensorBus/3 -> BusCreator/3  "OBJ_ID"
  SensorBus/2 -> BusCreator/2  "width"
  SensorBus/1 -> BusCreator/1  "time"
  BusCreator/1 -> SensorOut/1

== system First_HIL_Scenario2/Veh_1/Sensors/RadarSensor.3 ==
  BusCreator : BusCreator  Inputs=time,width,OBJ_ID,OBJ_Class,OBJ_S_Azimuth,OBJ_S_Elevation,OBJ_S_Velocity,OBJ_S_Range,OBJ_RCS
  SensorBus : S-Function  FunctionName=DataReceiver  Parameters='RadarSensor.3','time@i,64@[,OBJ_ID@i,OBJ_Class@i,OBJ_S_Azimuth@d,OBJ_S_Elevation@d,OBJ_S_Velocity@d,OBJ_S_Range@d,OBJ_RCS@d','0.01','0.0','192.168.2.195','25109'  SFunctionDeploymentMode=off  EnableBusSupport=off
  SensorOut : Outport
  wires:
  SensorBus/9 -> BusCreator/9  "OBJ_RCS"
  SensorBus/8 -> BusCreator/8  "OBJ_S_Range"
  SensorBus/7 -> BusCreator/7  "OBJ_S_Velocity"
  SensorBus/6 -> BusCreator/6  "OBJ_S_Elevation"
  SensorBus/5 -> BusCreator/5  "OBJ_S_Azimuth"
  SensorBus/4 -> BusCreator/4  "OBJ_Class"
  SensorBus/3 -> BusCreator/3  "OBJ_ID"
  SensorBus/2 -> BusCreator/2  "width"
  SensorBus/1 -> BusCreator/1  "time"
  BusCreator/1 -> SensorOut/1

== system First_HIL_Scenario2/Veh_1/Sensors/RadarSensor.4 ==
  BusCreator : BusCreator  Inputs=time,width,OBJ_ID,OBJ_Class,OBJ_S_Azimuth,OBJ_S_Elevation,OBJ_S_Velocity,OBJ_S_Range,OBJ_RCS
  SensorBus : S-Function  FunctionName=DataReceiver  Parameters='RadarSensor.4','time@i,64@[,OBJ_ID@i,OBJ_Class@i,OBJ_S_Azimuth@d,OBJ_S_Elevation@d,OBJ_S_Velocity@d,OBJ_S_Range@d,OBJ_RCS@d','0.01','0.0','192.168.2.195','25110'  SFunctionDeploymentMode=off  EnableBusSupport=off
  SensorOut : Outport
  wires:
  SensorBus/9 -> BusCreator/9  "OBJ_RCS"
  SensorBus/8 -> BusCreator/8  "OBJ_S_Range"
  SensorBus/7 -> BusCreator/7  "OBJ_S_Velocity"
  SensorBus/6 -> BusCreator/6  "OBJ_S_Elevation"
  SensorBus/5 -> BusCreator/5  "OBJ_S_Azimuth"
  SensorBus/4 -> BusCreator/4  "OBJ_Class"
  SensorBus/3 -> BusCreator/3  "OBJ_ID"
  SensorBus/2 -> BusCreator/2  "width"
  SensorBus/1 -> BusCreator/1  "time"
  BusCreator/1 -> SensorOut/1

== system First_HIL_Scenario2/Veh_1/Sensors/TrafficLightPerception.0 ==
  BusCreator : BusCreator  Inputs=Timestamp,width,TrafficLight_Direction,TrafficLight_State,TrafficLight_Timer
  SensorBus : S-Function  FunctionName=DataReceiver  Parameters='TrafficLightPerception.0','Timestamp@i,4@[,TrafficLight_Direction@b,TrafficLight_State@b,TrafficLight_Timer@i','0.01','0.0','192.168.2.195','25104'  SFunctionDeploymentMode=off  EnableBusSupport=off
  SensorOut : Outport
  wires:
  SensorBus/5 -> BusCreator/5  "TrafficLight_Timer"
  SensorBus/4 -> BusCreator/4  "TrafficLight_State"
  SensorBus/3 -> BusCreator/3  "TrafficLight_Direction"
  SensorBus/2 -> BusCreator/2  "width"
  SensorBus/1 -> BusCreator/1  "Timestamp"
  BusCreator/1 -> SensorOut/1

== system First_HIL_Scenario2/Veh_1/Sensors/UltrasonicSensor.0 ==
  BusCreator : BusCreator  Inputs=time,width,distance
  SensorBus : S-Function  FunctionName=DataReceiver  Parameters='UltrasonicSensor.0','time@i,1@[,distance@d','0.01','0.0','192.168.2.195','25115'  SFunctionDeploymentMode=off  EnableBusSupport=off
  SensorOut : Outport
  wires:
  SensorBus/3 -> BusCreator/3  "distance"
  SensorBus/2 -> BusCreator/2  "width"
  SensorBus/1 -> BusCreator/1  "time"
  BusCreator/1 -> SensorOut/1

== system First_HIL_Scenario2/Veh_1/Sensors/UltrasonicSensor.1 ==
  BusCreator : BusCreator  Inputs=time,width,distance
  SensorBus : S-Function  FunctionName=DataReceiver  Parameters='UltrasonicSensor.1','time@i,1@[,distance@d','0.01','0.0','192.168.2.195','25116'  SFunctionDeploymentMode=off  EnableBusSupport=off
  SensorOut : Outport
  wires:
  SensorBus/3 -> BusCreator/3  "distance"
  SensorBus/2 -> BusCreator/2  "width"
  SensorBus/1 -> BusCreator/1  "time"
  BusCreator/1 -> SensorOut/1

== system First_HIL_Scenario2/Veh_1/Sensors/UltrasonicSensor.10 ==
  BusCreator : BusCreator  Inputs=time,width,distance
  SensorBus : S-Function  FunctionName=DataReceiver  Parameters='UltrasonicSensor.10','time@i,1@[,distance@d','0.01','0.0','192.168.2.195','25125'  SFunctionDeploymentMode=off  EnableBusSupport=off
  SensorOut : Outport
  wires:
  SensorBus/3 -> BusCreator/3  "distance"
  SensorBus/2 -> BusCreator/2  "width"
  SensorBus/1 -> BusCreator/1  "time"
  BusCreator/1 -> SensorOut/1

== system First_HIL_Scenario2/Veh_1/Sensors/UltrasonicSensor.11 ==
  BusCreator : BusCreator  Inputs=time,width,distance
  SensorBus : S-Function  FunctionName=DataReceiver  Parameters='UltrasonicSensor.11','time@i,1@[,distance@d','0.01','0.0','192.168.2.195','25126'  SFunctionDeploymentMode=off  EnableBusSupport=off
  SensorOut : Outport
  wires:
  SensorBus/3 -> BusCreator/3  "distance"
  SensorBus/2 -> BusCreator/2  "width"
  SensorBus/1 -> BusCreator/1  "time"
  BusCreator/1 -> SensorOut/1

== system First_HIL_Scenario2/Veh_1/Sensors/UltrasonicSensor.2 ==
  BusCreator : BusCreator  Inputs=time,width,distance
  SensorBus : S-Function  FunctionName=DataReceiver  Parameters='UltrasonicSensor.2','time@i,1@[,distance@d','0.01','0.0','192.168.2.195','25117'  SFunctionDeploymentMode=off  EnableBusSupport=off
  SensorOut : Outport
  wires:
  SensorBus/3 -> BusCreator/3  "distance"
  SensorBus/2 -> BusCreator/2  "width"
  SensorBus/1 -> BusCreator/1  "time"
  BusCreator/1 -> SensorOut/1

== system First_HIL_Scenario2/Veh_1/Sensors/UltrasonicSensor.3 ==
  BusCreator : BusCreator  Inputs=time,width,distance
  SensorBus : S-Function  FunctionName=DataReceiver  Parameters='UltrasonicSensor.3','time@i,1@[,distance@d','0.01','0.0','192.168.2.195','25118'  SFunctionDeploymentMode=off  EnableBusSupport=off
  SensorOut : Outport
  wires:
  SensorBus/3 -> BusCreator/3  "distance"
  SensorBus/2 -> BusCreator/2  "width"
  SensorBus/1 -> BusCreator/1  "time"
  BusCreator/1 -> SensorOut/1

== system First_HIL_Scenario2/Veh_1/Sensors/UltrasonicSensor.4 ==
  BusCreator : BusCreator  Inputs=time,width,distance
  SensorBus : S-Function  FunctionName=DataReceiver  Parameters='UltrasonicSensor.4','time@i,1@[,distance@d','0.01','0.0','192.168.2.195','25119'  SFunctionDeploymentMode=off  EnableBusSupport=off
  SensorOut : Outport
  wires:
  SensorBus/3 -> BusCreator/3  "distance"
  SensorBus/2 -> BusCreator/2  "width"
  SensorBus/1 -> BusCreator/1  "time"
  BusCreator/1 -> SensorOut/1

== system First_HIL_Scenario2/Veh_1/Sensors/UltrasonicSensor.5 ==
  BusCreator : BusCreator  Inputs=time,width,distance
  SensorBus : S-Function  FunctionName=DataReceiver  Parameters='UltrasonicSensor.5','time@i,1@[,distance@d','0.01','0.0','192.168.2.195','25120'  SFunctionDeploymentMode=off  EnableBusSupport=off
  SensorOut : Outport
  wires:
  SensorBus/3 -> BusCreator/3  "distance"
  SensorBus/2 -> BusCreator/2  "width"
  SensorBus/1 -> BusCreator/1  "time"
  BusCreator/1 -> SensorOut/1

== system First_HIL_Scenario2/Veh_1/Sensors/UltrasonicSensor.6 ==
  BusCreator : BusCreator  Inputs=time,width,distance
  SensorBus : S-Function  FunctionName=DataReceiver  Parameters='UltrasonicSensor.6','time@i,1@[,distance@d','0.01','0.0','192.168.2.195','25121'  SFunctionDeploymentMode=off  EnableBusSupport=off
  SensorOut : Outport
  wires:
  SensorBus/3 -> BusCreator/3  "distance"
  SensorBus/2 -> BusCreator/2  "width"
  SensorBus/1 -> BusCreator/1  "time"
  BusCreator/1 -> SensorOut/1

== system First_HIL_Scenario2/Veh_1/Sensors/UltrasonicSensor.7 ==
  BusCreator : BusCreator  Inputs=time,width,distance
  SensorBus : S-Function  FunctionName=DataReceiver  Parameters='UltrasonicSensor.7','time@i,1@[,distance@d','0.01','0.0','192.168.2.195','25122'  SFunctionDeploymentMode=off  EnableBusSupport=off
  SensorOut : Outport
  wires:
  SensorBus/3 -> BusCreator/3  "distance"
  SensorBus/2 -> BusCreator/2  "width"
  SensorBus/1 -> BusCreator/1  "time"
  BusCreator/1 -> SensorOut/1

== system First_HIL_Scenario2/Veh_1/Sensors/UltrasonicSensor.8 ==
  BusCreator : BusCreator  Inputs=time,width,distance
  SensorBus : S-Function  FunctionName=DataReceiver  Parameters='UltrasonicSensor.8','time@i,1@[,distance@d','0.01','0.0','192.168.2.195','25123'  SFunctionDeploymentMode=off  EnableBusSupport=off
  SensorOut : Outport
  wires:
  SensorBus/3 -> BusCreator/3  "distance"
  SensorBus/2 -> BusCreator/2  "width"
  SensorBus/1 -> BusCreator/1  "time"
  BusCreator/1 -> SensorOut/1

== system First_HIL_Scenario2/Veh_1/Sensors/UltrasonicSensor.9 ==
  BusCreator : BusCreator  Inputs=time,width,distance
  SensorBus : S-Function  FunctionName=DataReceiver  Parameters='UltrasonicSensor.9','time@i,1@[,distance@d','0.01','0.0','192.168.2.195','25124'  SFunctionDeploymentMode=off  EnableBusSupport=off
  SensorOut : Outport
  wires:
  SensorBus/3 -> BusCreator/3  "distance"
  SensorBus/2 -> BusCreator/2  "width"
  SensorBus/1 -> BusCreator/1  "time"
  BusCreator/1 -> SensorOut/1

== system First_HIL_Scenario2/Veh_1/Sensors/sensor_template ==
  BusCreator : BusCreator  Inputs=8
  SensorBus : S-Function  FunctionName=DataReceiver  Parameters='mmwradar.0','time@i,64@[,angle@d,distance@d,speed@d,type@b,energy@d,id@i','0.1','0.0','192.168.2.195','25100'  SFunctionDeploymentMode=off  EnableBusSupport=off
  SensorOut : Outport
  wires:
  BusCreator/1 -> SensorOut/1

== system First_HIL_Scenario2/Veh_1/VehicleDataBus/EgoBus ==
  clock : Inport
  VehiclleDyn : Inport  Port=2
  VehiclleDyn1 : Inport  Port=3
  VehiclleDyn2 : Inport  Port=4
  EgoDataBus : S-Function  FunctionName=DataSender  Parameters='ego','time@i,x@d,y@d,z@d,yaw@d,pitch@d,roll@d,vx@d','0.01','0.0','192.168.2.101','25001'  SFunctionDeploymentMode=off  EnableBusSupport=off
  VehBusSelector3 : BusSelector  Tag=PanoSim_System  OutputSignals=XO,YO,ZO,YAW,PITCH,ROLL,VX
  wires:
  VehBusSelector3/7 -> EgoDataBus/8  "<VX>"
  VehBusSelector3/6 -> EgoDataBus/7  "<ROLL>"
  VehBusSelector3/5 -> EgoDataBus/6  "<PITCH>"
  VehBusSelector3/4 -> EgoDataBus/5  "<YAW>"
  VehBusSelector3/3 -> EgoDataBus/4  "<ZO>"
  VehBusSelector3/2 -> EgoDataBus/3  "<YO>"
  VehBusSelector3/1 -> EgoDataBus/2  "<XO>"
  VehiclleDyn/1 -> VehBusSelector3/1
  clock/1 -> EgoDataBus/1

== system First_HIL_Scenario2/Veh_1/VehicleDataBus/EgoExtraBus ==
  clock : Inport
  VehiclleDyn : Inport  Port=2
  Constant : Constant
  EgoDataBusExtra : S-Function  FunctionName=DataSender  Parameters='ego','time@i,vx@d,vy@d,vz@d,avx@d,avy@d,avz@d,ax@d,ay@d,az@d,aax@d,aay@d,aaz@d','0.01','0.0','192.168.2.101','25003'  SFunctionDeploymentMode=off  EnableBusSupport=off
  VehBusSelector2 : BusSelector  Tag=PanoSim_System  OutputSignals=VX,VY,VZ,AVx,AVy,AVz,Ax,Ay,Az,AAx,AAy,AAz
  Out1 : Outport
  wires:
  clock/1 -> EgoDataBusExtra/1
  VehiclleDyn/1 -> VehBusSelector2/1
  VehBusSelector2/1 -> EgoDataBusExtra/2  "<VX>"
  VehBusSelector2/2 -> EgoDataBusExtra/3  "<VY>"
  VehBusSelector2/3 -> EgoDataBusExtra/4  "<VZ>"
  VehBusSelector2/4 -> EgoDataBusExtra/5  "<AVx>"
  VehBusSelector2/5 -> EgoDataBusExtra/6  "<AVy>"
  VehBusSelector2/6 -> EgoDataBusExtra/7  "<AVz>"
  VehBusSelector2/7 -> EgoDataBusExtra/8  "<Ax>"
  VehBusSelector2/8 -> EgoDataBusExtra/9  "<Ay>"
  VehBusSelector2/9 -> EgoDataBusExtra/10  "<Az>"
  VehBusSelector2/10 -> EgoDataBusExtra/11  "<AAx>"
  VehBusSelector2/11 -> EgoDataBusExtra/12  "<AAy>"
  VehBusSelector2/12 -> EgoDataBusExtra/13  "<AAz>"
  Constant/1 -> Out1/1

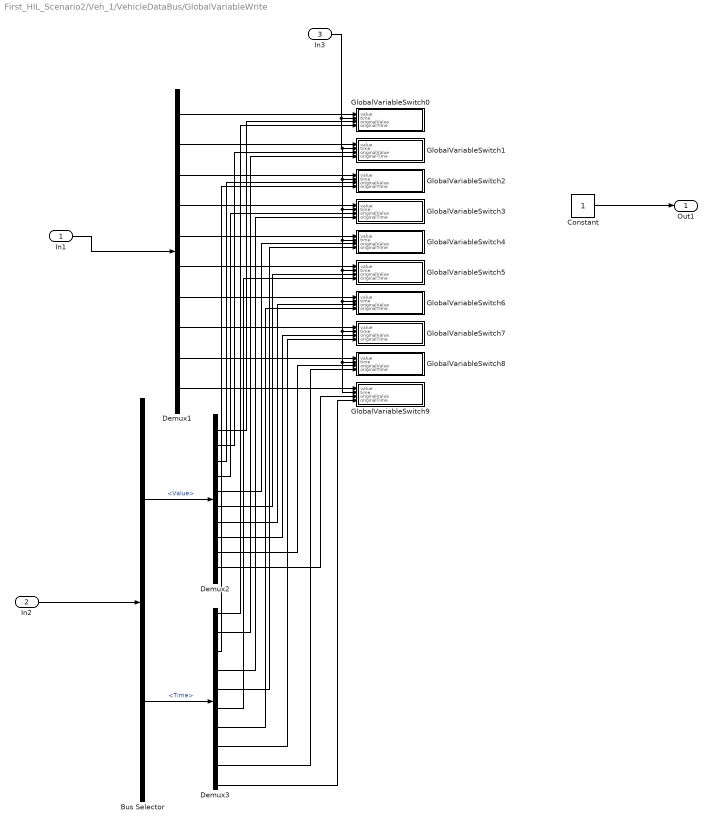
== system First_HIL_Scenario2/Veh_1/VehicleDataBus/GlobalVariableWrite ==
  In1 : Inport
  In2 : Inport  Port=2
  In3 : Inport  Port=3
  Bus Selector : BusSelector  OutputSignals=Value,Time
  Constant : Constant
  Demux1 : Demux  Outputs=10
  Demux2 : Demux  Outputs=10
  Demux3 : Demux  Outputs=10
  GlobalVariableSwitch0 : Subsystem
  GlobalVariableSwitch1 : Subsystem
  GlobalVariableSwitch2 : Subsystem
  GlobalVariableSwitch3 : Subsystem
  GlobalVariableSwitch4 : Subsystem
  GlobalVariableSwitch5 : Subsystem
  GlobalVariableSwitch6 : Subsystem
  GlobalVariableSwitch7 : Subsystem
  GlobalVariableSwitch8 : Subsystem
  GlobalVariableSwitch9 : Subsystem
  Out1 : Outport
  wires:
  Constant/1 -> Out1/1
  Demux3/10 -> GlobalVariableSwitch9/4(originalTIme)
  Demux2/10 -> GlobalVariableSwitch9/3(originalValue)
  Demux1/10 -> GlobalVariableSwitch9/1(value)
  Demux3/9 -> GlobalVariableSwitch8/4(originalTIme)
  Demux2/9 -> GlobalVariableSwitch8/3(originalValue)
  Demux1/9 -> GlobalVariableSwitch8/1(value)
  Demux3/8 -> GlobalVariableSwitch7/4(originalTIme)
  Demux2/8 -> GlobalVariableSwitch7/3(originalValue)
  Demux1/8 -> GlobalVariableSwitch7/1(value)
  Demux3/7 -> GlobalVariableSwitch6/4(originalTIme)
  Demux2/7 -> GlobalVariableSwitch6/3(originalValue)
  Demux1/7 -> GlobalVariableSwitch6/1(value)
  Demux3/6 -> GlobalVariableSwitch5/4(originalTIme)
  Demux2/6 -> GlobalVariableSwitch5/3(originalValue)
  Demux1/6 -> GlobalVariableSwitch5/1(value)
  Demux3/5 -> GlobalVariableSwitch4/4(originalTIme)
  Demux2/5 -> GlobalVariableSwitch4/3(originalValue)
  Demux1/5 -> GlobalVariableSwitch4/1(value)
  Demux3/4 -> GlobalVariableSwitch3/4(originalTIme)
  Demux2/4 -> GlobalVariableSwitch3/3(originalValue)
  Demux1/4 -> GlobalVariableSwitch3/1(value)
  Demux2/3 -> GlobalVariableSwitch2/3(originalValue)
  Demux3/3 -> GlobalVariableSwitch2/4(originalTIme)
  Demux1/3 -> GlobalVariableSwitch2/1(value)
  Demux3/2 -> GlobalVariableSwitch1/4(originalTIme)
  Demux2/2 -> GlobalVariableSwitch1/3(originalValue)
  Demux1/2 -> GlobalVariableSwitch1/1(value)
  Demux3/1 -> GlobalVariableSwitch0/4(originalTIme)
  Demux2/1 -> GlobalVariableSwitch0/3(originalValue)
  Bus Selector/2 -> Demux3/1  "<Time>"
  Bus Selector/1 -> Demux2/1  "<Value>"
  In3/1 -> GlobalVariableSwitch0/2(time), GlobalVariableSwitch1/2(time), GlobalVariableSwitch2/2(time), GlobalVariableSwitch3/2(time), GlobalVariableSwitch4/2(time), GlobalVariableSwitch5/2(time), GlobalVariableSwitch6/2(time), GlobalVariableSwitch7/2(time), GlobalVariableSwitch8/2(time), GlobalVariableSwitch9/2(time)
  Demux1/1 -> GlobalVariableSwitch0/1(value)
  In2/1 -> Bus Selector/1
  In1/1 -> Demux1/1

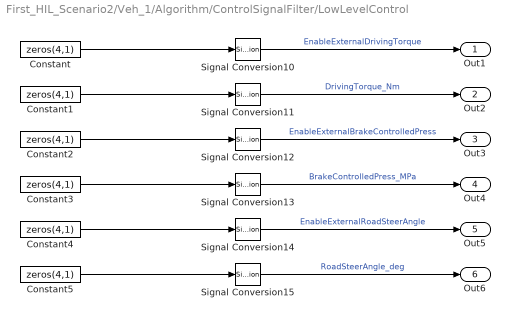
== system First_HIL_Scenario2/Veh_1/Algorithm/ControlSignalFilter/LowLevelControl ==
  Constant{,1..5} (6 alike) : Constant  Value=zeros(4,1)
  Signal Conversion{10..15} (6 alike) : SignalConversion  OverrideOpt=off
  Out1 : Outport
  Out2 : Outport  Port=2
  Out3 : Outport  Port=3
  Out4 : Outport  Port=4
  Out5 : Outport  Port=5
  Out6 : Outport  Port=6
  wires:
  Signal Conversion14/1 -> Out5/1  "EnableExternalRoadSteerAngle"
  Constant2/1 -> Signal Conversion12/1
  Constant3/1 -> Signal Conversion13/1
  Constant5/1 -> Signal Conversion15/1
  Signal Conversion10/1 -> Out1/1  "EnableExternalDrivingTorque"
  Constant/1 -> Signal Conversion10/1
  Constant1/1 -> Signal Conversion11/1
  Signal Conversion12/1 -> Out3/1  "EnableExternalBrakeControlledPress"
  Signal Conversion13/1 -> Out4/1  "BrakeControlledPress_MPa"
  Signal Conversion11/1 -> Out2/1  "DrivingTorque_Nm"
  Constant4/1 -> Signal Conversion14/1
  Signal Conversion15/1 -> Out6/1  "RoadSteerAngle_deg"

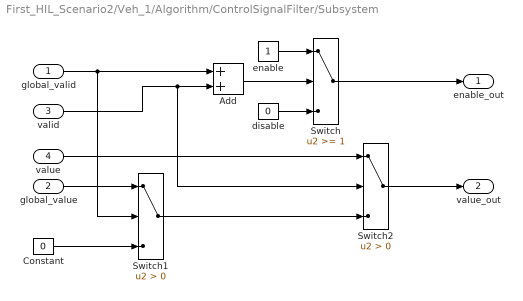
== system First_HIL_Scenario2/Veh_1/Algorithm/ControlSignalFilter/Subsystem ==
  global_valid : Inport
  global_value : Inport  Port=2
  valid : Inport  Port=3
  value : Inport  Port=4
  Add : Sum
  Constant : Constant  Value=0
  Switch : Switch  Threshold=1  SaturateOnIntegerOverflow=off  InputSameDT=off
  Switch1 : Switch  Criteria=u2 > Threshold  SaturateOnIntegerOverflow=off  InputSameDT=off
  Switch2 : Switch  Criteria=u2 > Threshold  SaturateOnIntegerOverflow=off  InputSameDT=off
  disable : Constant  Value=0
  enable : Constant
  enable_out : Outport
  value_out : Outport  Port=2
  wires:
  global_valid/1 -> Switch1/2, Add/1
  valid/1 -> Switch2/2, Add/2
  Add/1 -> Switch/2
  enable/1 -> Switch/1
  disable/1 -> Switch/3
  Switch/1 -> enable_out/1
  global_value/1 -> Switch1/1
  value/1 -> Switch2/1
  Constant/1 -> Switch1/3
  Switch1/1 -> Switch2/3
  Switch2/1 -> value_out/1

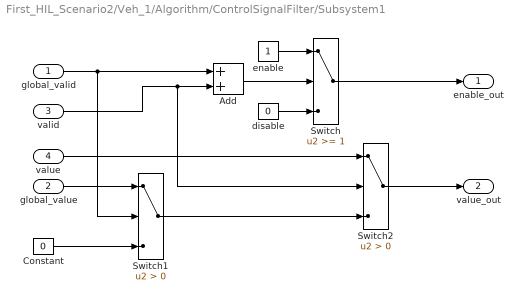
== system First_HIL_Scenario2/Veh_1/Algorithm/ControlSignalFilter/Subsystem1 ==
  global_valid : Inport
  global_value : Inport  Port=2
  valid : Inport  Port=3
  value : Inport  Port=4
  Add : Sum
  Constant : Constant  Value=0
  Switch : Switch  Threshold=1  SaturateOnIntegerOverflow=off  InputSameDT=off
  Switch1 : Switch  Criteria=u2 > Threshold  SaturateOnIntegerOverflow=off  InputSameDT=off
  Switch2 : Switch  Criteria=u2 > Threshold  SaturateOnIntegerOverflow=off  InputSameDT=off
  disable : Constant  Value=0
  enable : Constant
  enable_out : Outport
  value_out : Outport  Port=2
  wires:
  global_valid/1 -> Switch1/2, Add/1
  valid/1 -> Switch2/2, Add/2
  Add/1 -> Switch/2
  enable/1 -> Switch/1
  disable/1 -> Switch/3
  Switch/1 -> enable_out/1
  global_value/1 -> Switch1/1
  value/1 -> Switch2/1
  Constant/1 -> Switch1/3
  Switch1/1 -> Switch2/3
  Switch2/1 -> value_out/1

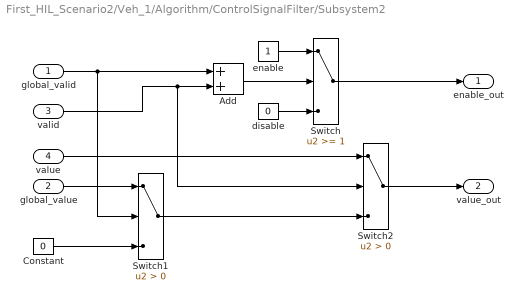
== system First_HIL_Scenario2/Veh_1/Algorithm/ControlSignalFilter/Subsystem2 ==
  global_valid : Inport
  global_value : Inport  Port=2
  valid : Inport  Port=3
  value : Inport  Port=4
  Add : Sum
  Constant : Constant  Value=0
  Switch : Switch  Threshold=1  SaturateOnIntegerOverflow=off  InputSameDT=off
  Switch1 : Switch  Criteria=u2 > Threshold  SaturateOnIntegerOverflow=off  InputSameDT=off
  Switch2 : Switch  Criteria=u2 > Threshold  SaturateOnIntegerOverflow=off  InputSameDT=off
  disable : Constant  Value=0
  enable : Constant
  enable_out : Outport
  value_out : Outport  Port=2
  wires:
  global_valid/1 -> Switch1/2, Add/1
  valid/1 -> Switch2/2, Add/2
  Add/1 -> Switch/2
  enable/1 -> Switch/1
  disable/1 -> Switch/3
  Switch/1 -> enable_out/1
  global_value/1 -> Switch1/1
  value/1 -> Switch2/1
  Constant/1 -> Switch1/3
  Switch1/1 -> Switch2/3
  Switch2/1 -> value_out/1
